simulink model "DCDC_SEPIC_Efficiency_Analysis"  (R2021b)
settings: Solver=ode23t  StartTime=0.0  StopTime=2  RelTol=1e-3
undefined symbols (not defined in the file): desired_dcMax, desiredCurrent_Param, desiredLoad_Param, desiredVoltage_Param, psu_V
libraries: fl_lib x5, nesl_utility x4, simulink x4, slpidlib x1, ee_lib x1
settings Model: Creator=vlenzi  LastModifiedBy=vlenzi
settings DataIOCC: SaveOutput=off  SignalLogging=off  DSMLogging=off  SaveTime=off
settings SimscapeCC: SimscapeLogType=all

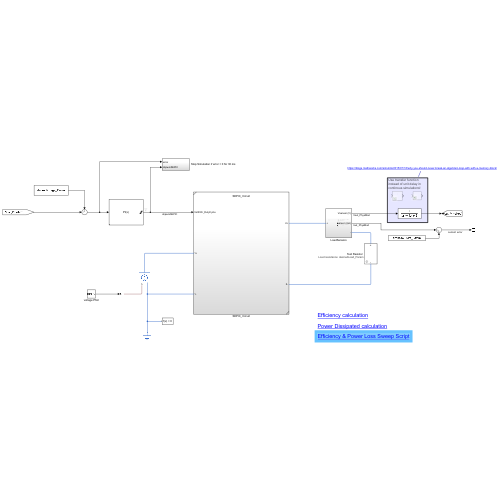
[thumbnail: Simulink's stored preview of the top-level diagram]
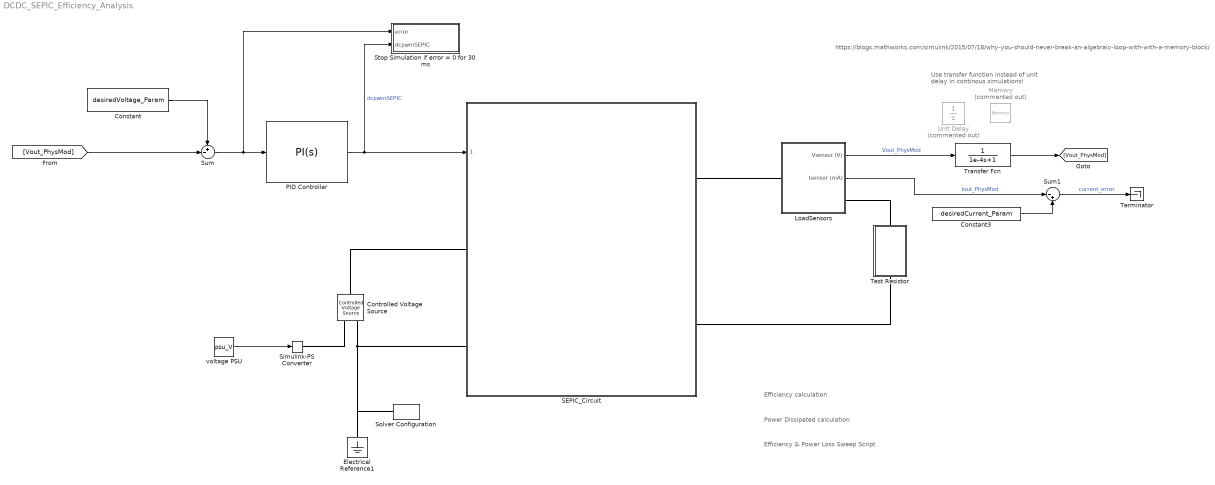
== system DCDC_SEPIC_Efficiency_Analysis ==
  note: https://blogs.mathworks.com/simulink/2015/07/18/why-you-should-never-break-an-algebraic-loop-with-with-a-memory-block/
  note: Efficiency calculation
  note: Power Dissipated calculation
  note: Efficiency & Power Loss Sweep Script
  note: Use transfer function
      | instead of unit delay in
      | continous simulations!
  Constant : Constant  Value=desiredVoltage_Param
  Constant3 : Constant  Value=desiredCurrent_Param
  Controlled Voltage Source : fl_lib/Electrical/Electrical Sources/Controlled Voltage Source
  Electrical Reference1 : fl_lib/Electrical/Electrical Elements/Electrical Reference
  LoadSensors : Subsystem
  Memory : Memory  Commented=on
  PID Controller : slpidlib/PID Controller  Controller=PI  Form=Parallel  TimeDomain=Continuous-time  UseExternalTs=off  SampleTime=1e-4  IntegratorMethod=Forward Euler  FilterMethod=Forward Euler  ControllerParametersSource=internal  P=0.1  I=2  D=0  UseFilter=on  N=100  TunerSelectOption=Transfer Function Based (PID Tuner App)  ZeroCross=off  InitialConditionSource=internal  InitialConditionForIntegrator=0  InitialConditionForFilter=0  DifferentiatorICPrevScaledInput=0  ExternalReset=none  TrackingMode=off  Kt=1  LimitOutput=on  SatLimitsSource=internal  UpperSaturationLimit=desired_dcMax  LowerSaturationLimit=0.0  LinearizeAsGain=on  AntiWindupMode=clamping  Kb=1  POutMin=[]  POutMax=[]  IOutMin=[]  IOutMax=[]  DOutMin=[]  DOutMax=[]  NOutMin=[]  NOutMax=[]  SumOutMin=[]  SumOutMax=[]  SaturationOutMin=[]  SaturationOutMax=[]  PParamMin=[]  PParamMax=[]  IParamMin=[]  IParamMax=[]  DParamMin=[]  DParamMax=[]  NParamMin=[]  NParamMax=[]  KbParamMin=[]  KbParamMax=[]  KtParamMin=[]  KtParamMax=[]  KbOutMin=[]  KbOutMax=[]  KtOutMin=[]  KtOutMax=[]  IntegratorOutMin=[]  IntegratorOutMax=[]  FilterOutMin=[]  FilterOutMax=[]  SumI1OutMin=[]  SumI1OutMax=[]  SumI2OutMin=[]  SumI2OutMax=[]  SumI3OutMin=[]  SumI3OutMax=[]  SumI4OutMin=[]  SumI4OutMax=[]  SumDOutMin=[]  SumDOutMax=[]  DifferentiatorOutMin=[]  DifferentiatorOutMax=[]  FilterDiffOutCoefMin=[]  FilterDiffOutCoefMax=[]  ReciprocalOutMin=[]  ReciprocalOutMax=[]  SumDenOutMin=[]  SumDenOutMax=[]  SumNumOutMin=[]  SumNumOutMax=[]  DivideOutMin=[]  DivideOutMax=[]  UdiffTsProdOutMin=[]  UdiffTsProdOutMax=[]  NTsProdOutMin=[]  NTsProdOutMax=[]  UintegralTsProdOutMin=[]  UintegralTsProdOutMax=[]  UngainTsProdOutMin=[]  UngainTsProdOutMax=[]  IntegratorContinuousStateAttributes=''  IntegratorStateMustResolveToSignalObject=off  IntegratorRTWStateStorageClass=Auto  FilterContinuousStateAttributes=''  FilterStateMustResolveToSignalObject=off  FilterRTWStateStorageClass=Auto  ParallelPVariant=InternalParameters  IdealPVariant=Disabled  IVariant=InternalParameters  DVariant=Disabled  IntegratorVariant=Continuous  SatVariant=Enabled  AWVariant=ContClampingParallel  PCopyVariant=Disabled  TRVariant=Disabled  FdbkBlocksVariant=Forward  IdealPFdbkVariant=Disabled  SatFdbkVariant=Disabled  DerivativeFilterVariant=Disabled  NVariant=Disabled  NCopyVariant=Disabled_SignalSpec  FilterICVariant=Disabled  IntegratorICVariant=InternalICs  ExternalResetVariant=Disabled  TRSumVariant=Passthrough  SumFdbkVariant=Disabled  SumVariant=Sum_PI  TsampFilterVariant=InternalTs  TsampNgainVariant=Passthrough  TsampIntegralVariant=Passthrough  ExternalSaturationOutDataTypeStr=Inherit: Same as second input
  SEPIC_Circuit : Subsystem  VariantControl=Var_Converter==2  ReferencedSubsystem=SEPIC_Circuit
  Simulink-PS Converter : nesl_utility/Simulink-PS Converter  PhysicalDomain=network_engine_domain  SubClassName=ps_input  LeftPortType=input  RightPortType=output  PseudoPeriodic=off  Frequencies=[]  NoiseDistribution=none  NoiseParameters=[]  Unit=V  AffineConversion=off  FilteringAndDerivatives=provide  SimscapeFilterOrder=1  InputFilterTimeConstant=0.001  UdotUserProvided=0
      settings: SourceProductBaseCode=PW,SS
  Solver Configuration : nesl_utility/Solver Configuration  PhysicalDomain=network_engine_domain  SubClassName=solver  LeftPortType=input  RightPortType=generic  Tones=[]  Harmonics=[]  SimulateNoise=off  Profile=off  UseLocalSampling=off  EnableSwitchedLinearOptims=on  FrequencyDomain=off  UseCCode=off  RelTol=0.001  AbsTol=1e-06  MinStep=1e-09  ToWorkspace=off  RevertToSquareIcSolve=off  NumHomotopyIterations=100  PhasorMode=off  PhasorModeNumHarmonics=1  DoDC=off  ResidualTolerance=1e-9  UseLocalSolver=off  LocalSolverChoice=NE_BACKWARD_EULER_ADVANCER  LocalSolverSampleTime=2e-7  DoFixedCost=off  MaxNonlinIter=2  MaxModeIter=2  ComputeImpulses=off  ImpulseIterations=2  LinearAlgebra=Sparse  EquationFormulation=NE_TIME_EF  DelaysMemoryBudget=1024  AutomaticFiltering=on  FilteringTimeConstant=0.001  PartitionStorageMethod=AS_NEEDED  PartitionMemoryBudget=1024  PartitionMethod=ROBUST
      settings: SourceProductBaseCode=PW,SS
  Stop Simulation if error = 0 for 30 ms : Subsystem
  Sum : Sum  Inputs=+-|
  Sum1 : Sum  Inputs=|-+
  Terminator : Terminator
  Test Resistor : Subsystem  VariantControl=Resistor  mask(Test Resistor){R_load=desiredLoad_Param, R_tol=1}
      mask prompts: R_load "Load Resistance [ohm]"; R_tol "Tolerance [%]"
      mask help: Test resistor with Load in the name, so that it can be triggered by ee_getEfficiency function.
      settings: AttributesFormatString=Load resistance: %<R_load>
  Transfer Fcn : TransferFcn  Denominator=[1e-4 1]
  Unit Delay : UnitDelay  Commented=on  SampleTime=-1  HasFrameUpgradeWarning=on
  voltage PSU : Constant  Value=psu_V  OutDataTypeStr=double
  wires:
  Constant/1 -> Sum/1
  PID Controller/1 -> SEPIC_Circuit/1, Stop Simulation if error = 0 for 30 ms/2(dcpwmSEPIC)  "dcpwmSEPIC"
  LoadSensors/1(Vsensor (V)) -> Transfer Fcn/1  "Vout_PhysMod"
  Sum/1 -> Stop Simulation if error = 0 for 30 ms/1(error), PID Controller/1
  voltage PSU/1 -> Simulink-PS Converter/1
  [Vout_PhysMod] -> Sum/2
  Transfer Fcn/1 -> [Vout_PhysMod]
  LoadSensors/2(Isensor (mA)) -> Sum1/1  "Iout_PhysMod"
  Sum1/1 -> Terminator/1  "current_error"
  Constant3/1 -> Sum1/2
  connections:
  Controlled Voltage Source/RConn2 -- Solver Configuration/RConn1 -- Electrical Reference1/LConn1 -- SEPIC_Circuit/LConn2
  Controlled Voltage Source/LConn1 -- SEPIC_Circuit/LConn1
  SEPIC_Circuit/RConn1 -- LoadSensors/LConn1
  Controlled Voltage Source/RConn1 -- Simulink-PS Converter/RConn1
  Test Resistor/LConn1 -- LoadSensors/RConn1
  SEPIC_Circuit/RConn2 -- Test Resistor/RConn1

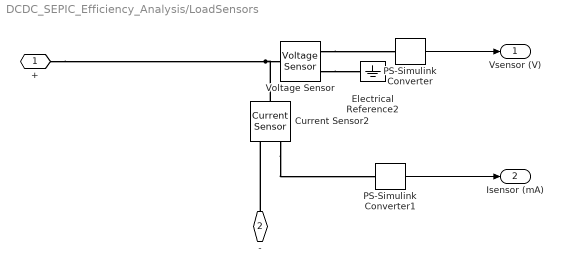
== system DCDC_SEPIC_Efficiency_Analysis/LoadSensors ==
  Current Sensor2 : fl_lib/Electrical/Electrical Sensors/Current Sensor
  Electrical Reference2 : fl_lib/Electrical/Electrical Elements/Electrical Reference
  PS-Simulink Converter : nesl_utility/PS-Simulink Converter  PhysicalDomain=network_engine_domain  SubClassName=ps_output  LeftPortType=input  RightPortType=output  PseudoPeriodic=off  Frequencies=[]  Unit=V  AffineConversion=off
      settings: SourceProductBaseCode=PW,SS
  PS-Simulink Converter1 : nesl_utility/PS-Simulink Converter  PhysicalDomain=network_engine_domain  SubClassName=ps_output  LeftPortType=input  RightPortType=output  PseudoPeriodic=off  Frequencies=[]  Unit=mA  AffineConversion=off
      settings: SourceProductBaseCode=PW,SS
  Voltage Sensor : fl_lib/Electrical/Electrical Sensors/Voltage Sensor
  + : PMIOPort  Side=Left
  - : PMIOPort  Port=2  Side=Right
  Vsensor (V) : Outport  Unit=V  VectorParamsAs1DForOutWhenUnconnected=off
  Isensor (mA) : Outport  Port=2  Unit=mA  VectorParamsAs1DForOutWhenUnconnected=off
  wires:
  PS-Simulink Converter/1 -> Vsensor (V)/1
  PS-Simulink Converter1/1 -> Isensor (mA)/1
  connections:
  -/RConn1 -- Current Sensor2/RConn2
  Current Sensor2/RConn1 -- PS-Simulink Converter1/LConn1
  +/RConn1 -- Voltage Sensor/LConn1 -- Current Sensor2/LConn1
  Voltage Sensor/RConn2 -- Electrical Reference2/LConn1
  Voltage Sensor/RConn1 -- PS-Simulink Converter/LConn1

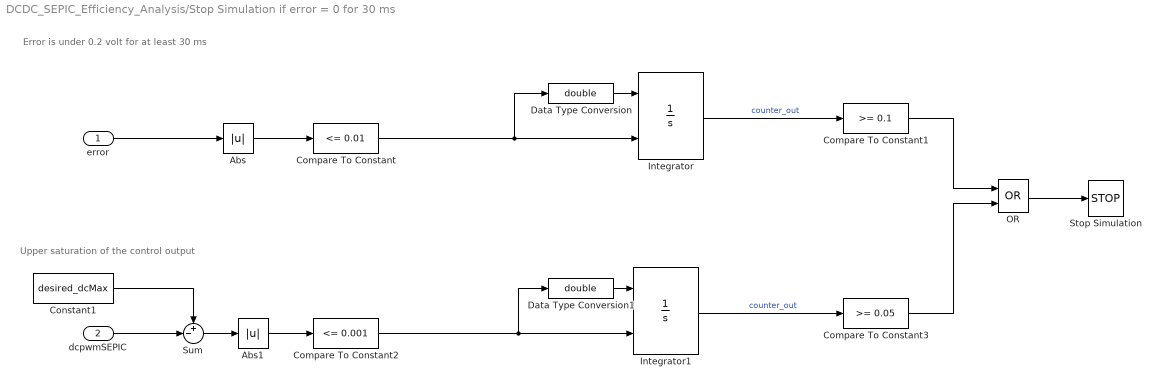
== system DCDC_SEPIC_Efficiency_Analysis/Stop Simulation if error = 0 for 30 ms ==
  note: Error is under 0.2 volt for at least 30 ms
  note: Upper saturation of the control output
  error : Inport
  dcpwmSEPIC : Inport  Port=2
  Abs : Abs
  Abs1 : Abs  ZeroCross=off
  Compare To Constant : simulink/Logic and Bit Operations/Compare To Constant  relop=<=  const=0.01  OutDataTypeStr=boolean
  Compare To Constant1 : simulink/Logic and Bit Operations/Compare To Constant  relop=>=  const=0.1  OutDataTypeStr=boolean
  Compare To Constant2 : simulink/Logic and Bit Operations/Compare To Constant  relop=<=  const=0.001  OutDataTypeStr=boolean
  Compare To Constant3 : simulink/Logic and Bit Operations/Compare To Constant  relop=>=  const=0.05  OutDataTypeStr=boolean
  Constant1 : Constant  Value=desired_dcMax
  Data Type Conversion : DataTypeConversion  OutDataTypeStr=double
  Data Type Conversion1 : DataTypeConversion  OutDataTypeStr=double
  Integrator : Integrator  ExternalReset=rising
  Integrator1 : Integrator  ExternalReset=rising
  OR : Logic  Operator=OR  AllPortsSameDT=off  OutDataTypeStr=boolean
  Stop Simulation : Stop
  Sum : Sum  Inputs=+-|
  wires:
  error/1 -> Abs/1
  Abs/1 -> Compare To Constant/1
  Integrator/1 -> Compare To Constant1/1  "counter_out"
  Compare To Constant/1 -> Data Type Conversion/1, Integrator/2
  Compare To Constant1/1 -> OR/1
  dcpwmSEPIC/1 -> Sum/2
  Constant1/1 -> Sum/1
  Sum/1 -> Abs1/1
  Abs1/1 -> Compare To Constant2/1
  Compare To Constant2/1 -> Data Type Conversion1/1, Integrator1/2
  Integrator1/1 -> Compare To Constant3/1  "counter_out"
  Compare To Constant3/1 -> OR/2
  OR/1 -> Stop Simulation/1
  Data Type Conversion/1 -> Integrator/1
  Data Type Conversion1/1 -> Integrator1/1

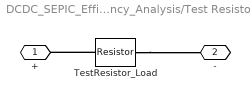
== system DCDC_SEPIC_Efficiency_Analysis/Test Resistor ==
  TestResistor_Load : ee_lib/Passive/Resistor  R=R_load Ohm  R_tol=R_tol  enable_R_tol=0  tol_distribution=1  nSigma=4  enable_operating_limits=0  operating_limit_action=2  max_working_voltage=100 V  power_rating=1 W  enable_faults=0  fault_action=1  R_faulted=inf Ohm  enable_temporal_fault=0  t_fault=1 s  enable_behavioral_fault=0  max_permissible_current=1 A  t_fail_on_current=1 s  noise_mode=0  sample_time=1e-3 s  repeatability=1  auto_seed=3536724442  user_seed=0  Tdevice=25 degC  power_derating_T1=70 degC  power_derating_T2=155 degC  operating_temperature_range_vec=[-50, 150] degC  alpha=3.93e-3 1/K  Tmeas=25 degC  thermal_mass=100 J/K  temperature_specify=off  temperature_priority=High  temperature=298.15 K  temperature_nominal_specify=off  temperature_nominal_unit=K  temperature_nominal_value=1
  + : PMIOPort  Side=Left
  - : PMIOPort  Port=2  Side=Right
  connections:
  TestResistor_Load/LConn1 -- +/RConn1
  TestResistor_Load/RConn1 -- -/RConn1
